simulink library "tramontina_database_xsenslib"  (R2023b)
settings: Solver=VariableStepAuto  StartTime=0.0  StopTime=10.0  RelTol=1e-3
libraries: canmsglib x46, simulink x1
(part 2 of 2)

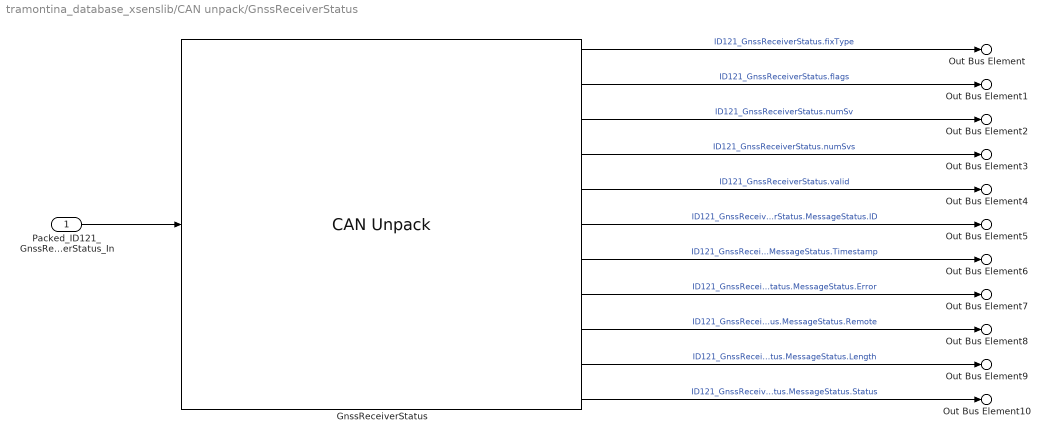
== system tramontina_database_xsenslib/CAN unpack/GnssReceiverStatus ==
  Packed_ID121_GnssReceiverStatus_In : Inport
  GnssReceiverStatus : canmsglib/CAN Unpack  CANdbFile=C:\Users\matlab.cut\Desktop\AMR\canbus_files\tramontina_database_xsens.dbc  MsgList=GnssReceiverStatus  MsgName=GnssReceiverStatus  MsgIDType=Standard (11-bit identifier)  MsgIdentifier=121  MsgLength=5  SignalInfo={'fixType','0','8','BE','unsigned','Standard','0','1','0','-Inf','Inf';'flags','16','8','BE','unsigned','Standard','0','1','0','-Inf','Inf';'numSv','8','8','BE','unsigned','Standard','0','1','0','-Inf','Inf';'numSvs','32','8','BE','unsigned','Standard','0','1','1','-Inf','Inf';'valid','24','8','BE','unsigned','Standard','0','1','0','-Inf','Inf'}  IDPort=on  TimestampPort=on  ErrorPort=on  RemotePort=on  LengthPort=on  StatusPort=on  ApplyMinMax=off
  Out Bus Element : Outport  PortName=ID121_GnssReceiverStatus  Element=fixType
  Out Bus Element1 : Outport  PortName=ID121_GnssReceiverStatus  Element=flags
  Out Bus Element2 : Outport  PortName=ID121_GnssReceiverStatus  Element=numSv
  Out Bus Element3 : Outport  PortName=ID121_GnssReceiverStatus  Element=numSvs
  Out Bus Element4 : Outport  PortName=ID121_GnssReceiverStatus  Element=valid
  Out Bus Element5 : Outport  PortName=ID121_GnssReceiverStatus  Element=MessageStatus.ID
  Out Bus Element6 : Outport  PortName=ID121_GnssReceiverStatus  Element=MessageStatus.Timestamp
  Out Bus Element7 : Outport  PortName=ID121_GnssReceiverStatus  Element=MessageStatus.Error
  Out Bus Element8 : Outport  PortName=ID121_GnssReceiverStatus  Element=MessageStatus.Remote
  Out Bus Element9 : Outport  PortName=ID121_GnssReceiverStatus  Element=MessageStatus.Length
  Out Bus Element10 : Outport  PortName=ID121_GnssReceiverStatus  Element=MessageStatus.Status
  wires:
  Packed_ID121_GnssReceiverStatus_In/1 -> GnssReceiverStatus/1
  GnssReceiverStatus/1 -> Out Bus Element/1  "ID121_GnssReceiverStatus.fixType"
  GnssReceiverStatus/2 -> Out Bus Element1/1  "ID121_GnssReceiverStatus.flags"
  GnssReceiverStatus/3 -> Out Bus Element2/1  "ID121_GnssReceiverStatus.numSv"
  GnssReceiverStatus/4 -> Out Bus Element3/1  "ID121_GnssReceiverStatus.numSvs"
  GnssReceiverStatus/5 -> Out Bus Element4/1  "ID121_GnssReceiverStatus.valid"
  GnssReceiverStatus/6 -> Out Bus Element5/1  "ID121_GnssReceiverStatus.MessageStatus.ID"
  GnssReceiverStatus/7 -> Out Bus Element6/1  "ID121_GnssReceiverStatus.MessageStatus.Timestamp"
  GnssReceiverStatus/8 -> Out Bus Element7/1  "ID121_GnssReceiverStatus.MessageStatus.Error"
  GnssReceiverStatus/9 -> Out Bus Element8/1  "ID121_GnssReceiverStatus.MessageStatus.Remote"
  GnssReceiverStatus/10 -> Out Bus Element9/1  "ID121_GnssReceiverStatus.MessageStatus.Length"
  GnssReceiverStatus/11 -> Out Bus Element10/1  "ID121_GnssReceiverStatus.MessageStatus.Status"

== system tramontina_database_xsenslib/CAN unpack/GroupCounter ==
  Packed_ID6_GroupCounter_In : Inport
  GroupCounter : canmsglib/CAN Unpack  CANdbFile=C:\Users\matlab.cut\Desktop\AMR\canbus_files\tramontina_database_xsens.dbc  MsgList=GroupCounter  MsgName=GroupCounter  MsgIDType=Standard (11-bit identifier)  MsgIdentifier=6  MsgLength=2  SignalInfo={'Counter','8','16','BE','unsigned','Standard','0','1','0','-Inf','Inf'}  IDPort=on  TimestampPort=on  ErrorPort=on  RemotePort=on  LengthPort=on  StatusPort=on  ApplyMinMax=off
  Out Bus Element : Outport  PortName=ID6_GroupCounter  Element=Counter
  Out Bus Element1 : Outport  PortName=ID6_GroupCounter  Element=MessageStatus.ID
  Out Bus Element2 : Outport  PortName=ID6_GroupCounter  Element=MessageStatus.Timestamp
  Out Bus Element3 : Outport  PortName=ID6_GroupCounter  Element=MessageStatus.Error
  Out Bus Element4 : Outport  PortName=ID6_GroupCounter  Element=MessageStatus.Remote
  Out Bus Element5 : Outport  PortName=ID6_GroupCounter  Element=MessageStatus.Length
  Out Bus Element6 : Outport  PortName=ID6_GroupCounter  Element=MessageStatus.Status
  wires:
  Packed_ID6_GroupCounter_In/1 -> GroupCounter/1
  GroupCounter/1 -> Out Bus Element/1  "ID6_GroupCounter.Counter"
  GroupCounter/2 -> Out Bus Element1/1  "ID6_GroupCounter.MessageStatus.ID"
  GroupCounter/3 -> Out Bus Element2/1  "ID6_GroupCounter.MessageStatus.Timestamp"
  GroupCounter/4 -> Out Bus Element3/1  "ID6_GroupCounter.MessageStatus.Error"
  GroupCounter/5 -> Out Bus Element4/1  "ID6_GroupCounter.MessageStatus.Remote"
  GroupCounter/6 -> Out Bus Element5/1  "ID6_GroupCounter.MessageStatus.Length"
  GroupCounter/7 -> Out Bus Element6/1  "ID6_GroupCounter.MessageStatus.Status"

== system tramontina_database_xsenslib/CAN unpack/LongLat ==
  Packed_ID113_LongLat_In : Inport
  LongLat : canmsglib/CAN Unpack  CANdbFile=C:\Users\matlab.cut\Desktop\AMR\canbus_files\tramontina_database_xsens.dbc  MsgList=LongLat  MsgName=LongLat  MsgIDType=Standard (11-bit identifier)  MsgIdentifier=113  MsgLength=8  SignalInfo={'latitude','24','32','BE','signed','Standard','0','5.9605e-08','0','-90','90';'longitude','56','32','BE','signed','Standard','0','1.1921e-07','0','-180','180'}  IDPort=on  TimestampPort=on  ErrorPort=on  RemotePort=on  LengthPort=on  StatusPort=on  ApplyMinMax=off
  Out Bus Element : Outport  PortName=ID113_LongLat  Element=latitude
  Out Bus Element1 : Outport  PortName=ID113_LongLat  Element=longitude
  Out Bus Element2 : Outport  PortName=ID113_LongLat  Element=MessageStatus.ID
  Out Bus Element3 : Outport  PortName=ID113_LongLat  Element=MessageStatus.Timestamp
  Out Bus Element4 : Outport  PortName=ID113_LongLat  Element=MessageStatus.Error
  Out Bus Element5 : Outport  PortName=ID113_LongLat  Element=MessageStatus.Remote
  Out Bus Element6 : Outport  PortName=ID113_LongLat  Element=MessageStatus.Length
  Out Bus Element7 : Outport  PortName=ID113_LongLat  Element=MessageStatus.Status
  wires:
  Packed_ID113_LongLat_In/1 -> LongLat/1
  LongLat/1 -> Out Bus Element/1  "ID113_LongLat.latitude"
  LongLat/2 -> Out Bus Element1/1  "ID113_LongLat.longitude"
  LongLat/3 -> Out Bus Element2/1  "ID113_LongLat.MessageStatus.ID"
  LongLat/4 -> Out Bus Element3/1  "ID113_LongLat.MessageStatus.Timestamp"
  LongLat/5 -> Out Bus Element4/1  "ID113_LongLat.MessageStatus.Error"
  LongLat/6 -> Out Bus Element5/1  "ID113_LongLat.MessageStatus.Remote"
  LongLat/7 -> Out Bus Element6/1  "ID113_LongLat.MessageStatus.Length"
  LongLat/8 -> Out Bus Element7/1  "ID113_LongLat.MessageStatus.Status"

== system tramontina_database_xsenslib/CAN unpack/MagneticField ==
  Packed_ID65_MagneticField_In : Inport
  MagneticField : canmsglib/CAN Unpack  CANdbFile=C:\Users\matlab.cut\Desktop\AMR\canbus_files\tramontina_database_xsens.dbc  MsgList=MagneticField  MsgName=MagneticField  MsgIDType=Standard (11-bit identifier)  MsgIdentifier=65  MsgLength=6  SignalInfo={'magX','8','16','BE','signed','Standard','0','0.00097656','0','-32','32';'magY','24','16','BE','signed','Standard','0','0.00097656','0','-32','32';'magZ','40','16','BE','signed','Standard','0','0.00097656','0','-32','32'}  IDPort=on  TimestampPort=on  ErrorPort=on  RemotePort=on  LengthPort=on  StatusPort=on  ApplyMinMax=off
  Out Bus Element : Outport  PortName=ID65_MagneticField  Element=magX
  Out Bus Element1 : Outport  PortName=ID65_MagneticField  Element=magY
  Out Bus Element2 : Outport  PortName=ID65_MagneticField  Element=magZ
  Out Bus Element3 : Outport  PortName=ID65_MagneticField  Element=MessageStatus.ID
  Out Bus Element4 : Outport  PortName=ID65_MagneticField  Element=MessageStatus.Timestamp
  Out Bus Element5 : Outport  PortName=ID65_MagneticField  Element=MessageStatus.Error
  Out Bus Element6 : Outport  PortName=ID65_MagneticField  Element=MessageStatus.Remote
  Out Bus Element7 : Outport  PortName=ID65_MagneticField  Element=MessageStatus.Length
  Out Bus Element8 : Outport  PortName=ID65_MagneticField  Element=MessageStatus.Status
  wires:
  Packed_ID65_MagneticField_In/1 -> MagneticField/1
  MagneticField/1 -> Out Bus Element/1  "ID65_MagneticField.magX"
  MagneticField/2 -> Out Bus Element1/1  "ID65_MagneticField.magY"
  MagneticField/3 -> Out Bus Element2/1  "ID65_MagneticField.magZ"
  MagneticField/4 -> Out Bus Element3/1  "ID65_MagneticField.MessageStatus.ID"
  MagneticField/5 -> Out Bus Element4/1  "ID65_MagneticField.MessageStatus.Timestamp"
  MagneticField/6 -> Out Bus Element5/1  "ID65_MagneticField.MessageStatus.Error"
  MagneticField/7 -> Out Bus Element6/1  "ID65_MagneticField.MessageStatus.Remote"
  MagneticField/8 -> Out Bus Element7/1  "ID65_MagneticField.MessageStatus.Length"
  MagneticField/9 -> Out Bus Element8/1  "ID65_MagneticField.MessageStatus.Status"

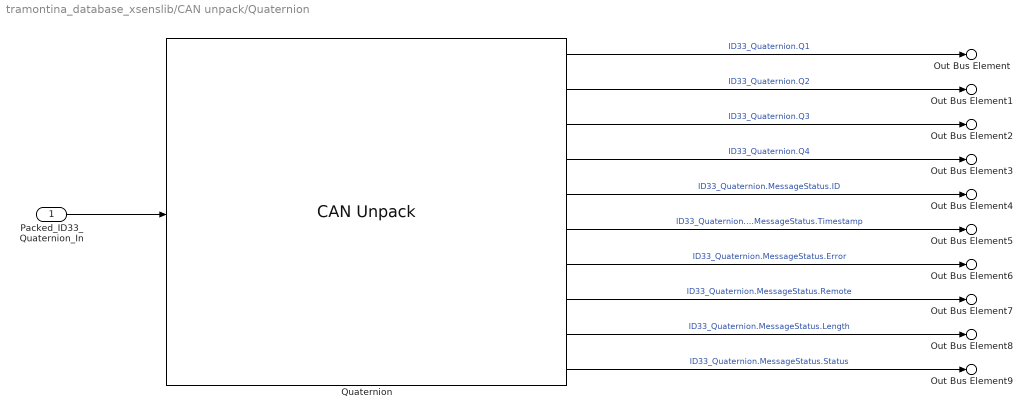
== system tramontina_database_xsenslib/CAN unpack/Quaternion ==
  Packed_ID33_Quaternion_In : Inport
  Quaternion : canmsglib/CAN Unpack  CANdbFile=C:\Users\matlab.cut\Desktop\AMR\canbus_files\tramontina_database_xsens.dbc  MsgList=Quaternion  MsgName=Quaternion  MsgIDType=Standard (11-bit identifier)  MsgIdentifier=33  MsgLength=8  SignalInfo={'Q1','8','16','BE','signed','Standard','0','3.0518e-05','0','-1','1';'Q2','24','16','BE','signed','Standard','0','3.0518e-05','0','-1','1';'Q3','40','16','BE','signed','Standard','0','3.0518e-05','0','-1','1';'Q4','56','16','BE','signed','Standard','0','3.0518e-05','0','-Inf','Inf'}  IDPort=on  TimestampPort=on  ErrorPort=on  RemotePort=on  LengthPort=on  StatusPort=on  ApplyMinMax=off
  Out Bus Element : Outport  PortName=ID33_Quaternion  Element=Q1
  Out Bus Element1 : Outport  PortName=ID33_Quaternion  Element=Q2
  Out Bus Element2 : Outport  PortName=ID33_Quaternion  Element=Q3
  Out Bus Element3 : Outport  PortName=ID33_Quaternion  Element=Q4
  Out Bus Element4 : Outport  PortName=ID33_Quaternion  Element=MessageStatus.ID
  Out Bus Element5 : Outport  PortName=ID33_Quaternion  Element=MessageStatus.Timestamp
  Out Bus Element6 : Outport  PortName=ID33_Quaternion  Element=MessageStatus.Error
  Out Bus Element7 : Outport  PortName=ID33_Quaternion  Element=MessageStatus.Remote
  Out Bus Element8 : Outport  PortName=ID33_Quaternion  Element=MessageStatus.Length
  Out Bus Element9 : Outport  PortName=ID33_Quaternion  Element=MessageStatus.Status
  wires:
  Packed_ID33_Quaternion_In/1 -> Quaternion/1
  Quaternion/1 -> Out Bus Element/1  "ID33_Quaternion.Q1"
  Quaternion/2 -> Out Bus Element1/1  "ID33_Quaternion.Q2"
  Quaternion/3 -> Out Bus Element2/1  "ID33_Quaternion.Q3"
  Quaternion/4 -> Out Bus Element3/1  "ID33_Quaternion.Q4"
  Quaternion/5 -> Out Bus Element4/1  "ID33_Quaternion.MessageStatus.ID"
  Quaternion/6 -> Out Bus Element5/1  "ID33_Quaternion.MessageStatus.Timestamp"
  Quaternion/7 -> Out Bus Element6/1  "ID33_Quaternion.MessageStatus.Error"
  Quaternion/8 -> Out Bus Element7/1  "ID33_Quaternion.MessageStatus.Remote"
  Quaternion/9 -> Out Bus Element8/1  "ID33_Quaternion.MessageStatus.Length"
  Quaternion/10 -> Out Bus Element9/1  "ID33_Quaternion.MessageStatus.Status"

== system tramontina_database_xsenslib/CAN unpack/RateOfTurn ==
  Packed_ID50_RateOfTurn_In : Inport
  RateOfTurn : canmsglib/CAN Unpack  CANdbFile=C:\Users\matlab.cut\Desktop\AMR\canbus_files\tramontina_database_xsens.dbc  MsgList=RateOfTurn  MsgName=RateOfTurn  MsgIDType=Standard (11-bit identifier)  MsgIdentifier=50  MsgLength=6  SignalInfo={'gyrX','8','16','BE','signed','Standard','0','0.0019531','0','-Inf','Inf';'gyrY','24','16','BE','signed','Standard','0','0.0019531','0','-Inf','Inf';'gyrZ','40','16','BE','signed','Standard','0','0.0019531','0','-Inf','Inf'}  IDPort=on  TimestampPort=on  ErrorPort=on  RemotePort=on  LengthPort=on  StatusPort=on  ApplyMinMax=off
  Out Bus Element : Outport  PortName=ID50_RateOfTurn  Element=gyrX
  Out Bus Element1 : Outport  PortName=ID50_RateOfTurn  Element=gyrY
  Out Bus Element2 : Outport  PortName=ID50_RateOfTurn  Element=gyrZ
  Out Bus Element3 : Outport  PortName=ID50_RateOfTurn  Element=MessageStatus.ID
  Out Bus Element4 : Outport  PortName=ID50_RateOfTurn  Element=MessageStatus.Timestamp
  Out Bus Element5 : Outport  PortName=ID50_RateOfTurn  Element=MessageStatus.Error
  Out Bus Element6 : Outport  PortName=ID50_RateOfTurn  Element=MessageStatus.Remote
  Out Bus Element7 : Outport  PortName=ID50_RateOfTurn  Element=MessageStatus.Length
  Out Bus Element8 : Outport  PortName=ID50_RateOfTurn  Element=MessageStatus.Status
  wires:
  Packed_ID50_RateOfTurn_In/1 -> RateOfTurn/1
  RateOfTurn/1 -> Out Bus Element/1  "ID50_RateOfTurn.gyrX"
  RateOfTurn/2 -> Out Bus Element1/1  "ID50_RateOfTurn.gyrY"
  RateOfTurn/3 -> Out Bus Element2/1  "ID50_RateOfTurn.gyrZ"
  RateOfTurn/4 -> Out Bus Element3/1  "ID50_RateOfTurn.MessageStatus.ID"
  RateOfTurn/5 -> Out Bus Element4/1  "ID50_RateOfTurn.MessageStatus.Timestamp"
  RateOfTurn/6 -> Out Bus Element5/1  "ID50_RateOfTurn.MessageStatus.Error"
  RateOfTurn/7 -> Out Bus Element6/1  "ID50_RateOfTurn.MessageStatus.Remote"
  RateOfTurn/8 -> Out Bus Element7/1  "ID50_RateOfTurn.MessageStatus.Length"
  RateOfTurn/9 -> Out Bus Element8/1  "ID50_RateOfTurn.MessageStatus.Status"

== system tramontina_database_xsenslib/CAN unpack/RateOfTurnHR ==
  Packed_ID97_RateOfTurnHR_In : Inport
  RateOfTurnHR : canmsglib/CAN Unpack  CANdbFile=C:\Users\matlab.cut\Desktop\AMR\canbus_files\tramontina_database_xsens.dbc  MsgList=RateOfTurnHR  MsgName=RateOfTurnHR  MsgIDType=Standard (11-bit identifier)  MsgIdentifier=97  MsgLength=6  SignalInfo={'HrGyrX','8','16','BE','signed','Standard','0','0.0019531','0','-Inf','Inf';'HrGyrY','24','16','BE','signed','Standard','0','0.0019531','0','-Inf','Inf';'HrGyrZ','40','16','BE','signed','Standard','0','0.0019531','0','-Inf','Inf'}  IDPort=on  TimestampPort=on  ErrorPort=on  RemotePort=on  LengthPort=on  StatusPort=on  ApplyMinMax=off
  Out Bus Element : Outport  PortName=ID97_RateOfTurnHR  Element=HrGyrX
  Out Bus Element1 : Outport  PortName=ID97_RateOfTurnHR  Element=HrGyrY
  Out Bus Element2 : Outport  PortName=ID97_RateOfTurnHR  Element=HrGyrZ
  Out Bus Element3 : Outport  PortName=ID97_RateOfTurnHR  Element=MessageStatus.ID
  Out Bus Element4 : Outport  PortName=ID97_RateOfTurnHR  Element=MessageStatus.Timestamp
  Out Bus Element5 : Outport  PortName=ID97_RateOfTurnHR  Element=MessageStatus.Error
  Out Bus Element6 : Outport  PortName=ID97_RateOfTurnHR  Element=MessageStatus.Remote
  Out Bus Element7 : Outport  PortName=ID97_RateOfTurnHR  Element=MessageStatus.Length
  Out Bus Element8 : Outport  PortName=ID97_RateOfTurnHR  Element=MessageStatus.Status
  wires:
  Packed_ID97_RateOfTurnHR_In/1 -> RateOfTurnHR/1
  RateOfTurnHR/1 -> Out Bus Element/1  "ID97_RateOfTurnHR.HrGyrX"
  RateOfTurnHR/2 -> Out Bus Element1/1  "ID97_RateOfTurnHR.HrGyrY"
  RateOfTurnHR/3 -> Out Bus Element2/1  "ID97_RateOfTurnHR.HrGyrZ"
  RateOfTurnHR/4 -> Out Bus Element3/1  "ID97_RateOfTurnHR.MessageStatus.ID"
  RateOfTurnHR/5 -> Out Bus Element4/1  "ID97_RateOfTurnHR.MessageStatus.Timestamp"
  RateOfTurnHR/6 -> Out Bus Element5/1  "ID97_RateOfTurnHR.MessageStatus.Error"
  RateOfTurnHR/7 -> Out Bus Element6/1  "ID97_RateOfTurnHR.MessageStatus.Remote"
  RateOfTurnHR/8 -> Out Bus Element7/1  "ID97_RateOfTurnHR.MessageStatus.Length"
  RateOfTurnHR/9 -> Out Bus Element8/1  "ID97_RateOfTurnHR.MessageStatus.Status"

== system tramontina_database_xsenslib/CAN unpack/SampleTime ==
  Packed_ID5_SampleTime_In : Inport
  SampleTime : canmsglib/CAN Unpack  CANdbFile=C:\Users\matlab.cut\Desktop\AMR\canbus_files\tramontina_database_xsens.dbc  MsgList=SampleTime  MsgName=SampleTime  MsgIDType=Standard (11-bit identifier)  MsgIdentifier=5  MsgLength=4  SignalInfo={'Timestamp','24','32','BE','unsigned','Standard','0','1','0','-Inf','Inf'}  IDPort=on  TimestampPort=on  ErrorPort=on  RemotePort=on  LengthPort=on  StatusPort=on  ApplyMinMax=off
  Out Bus Element : Outport  PortName=ID5_SampleTime  Element=Timestamp
  Out Bus Element1 : Outport  PortName=ID5_SampleTime  Element=MessageStatus.ID
  Out Bus Element2 : Outport  PortName=ID5_SampleTime  Element=MessageStatus.Timestamp
  Out Bus Element3 : Outport  PortName=ID5_SampleTime  Element=MessageStatus.Error
  Out Bus Element4 : Outport  PortName=ID5_SampleTime  Element=MessageStatus.Remote
  Out Bus Element5 : Outport  PortName=ID5_SampleTime  Element=MessageStatus.Length
  Out Bus Element6 : Outport  PortName=ID5_SampleTime  Element=MessageStatus.Status
  wires:
  Packed_ID5_SampleTime_In/1 -> SampleTime/1
  SampleTime/1 -> Out Bus Element/1  "ID5_SampleTime.Timestamp"
  SampleTime/2 -> Out Bus Element1/1  "ID5_SampleTime.MessageStatus.ID"
  SampleTime/3 -> Out Bus Element2/1  "ID5_SampleTime.MessageStatus.Timestamp"
  SampleTime/4 -> Out Bus Element3/1  "ID5_SampleTime.MessageStatus.Error"
  SampleTime/5 -> Out Bus Element4/1  "ID5_SampleTime.MessageStatus.Remote"
  SampleTime/6 -> Out Bus Element5/1  "ID5_SampleTime.MessageStatus.Length"
  SampleTime/7 -> Out Bus Element6/1  "ID5_SampleTime.MessageStatus.Status"

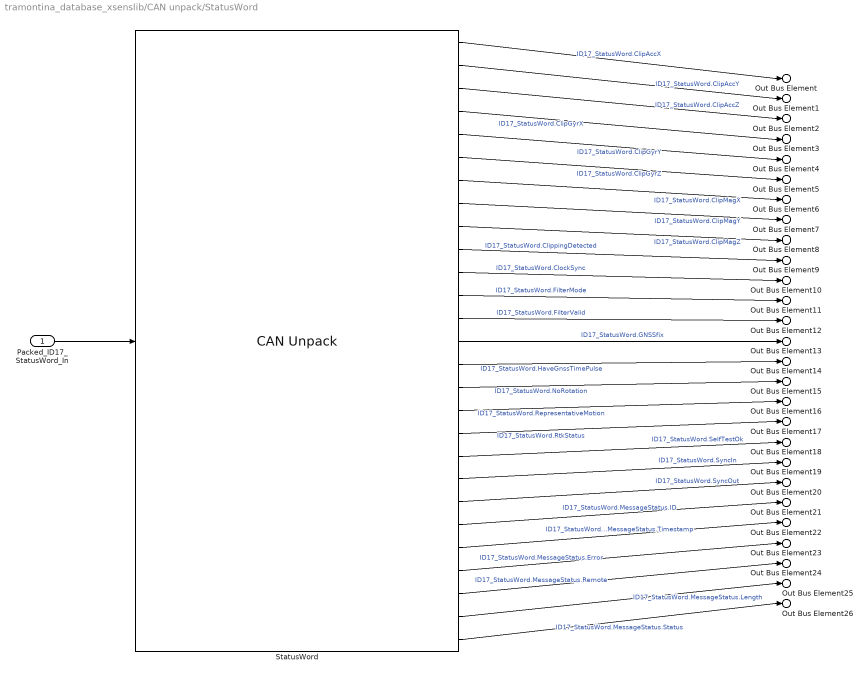
== system tramontina_database_xsenslib/CAN unpack/StatusWord ==
  Packed_ID17_StatusWord_In : Inport
  StatusWord : canmsglib/CAN Unpack  CANdbFile=C:\Users\matlab.cut\Desktop\AMR\canbus_files\tramontina_database_xsens.dbc  MsgList=StatusWord  MsgName=StatusWord  MsgIDType=Standard (11-bit identifier)  MsgIdentifier=17  MsgLength=4  SignalInfo={'ClipAccX','16','1','LE','unsigned','Standard','0','1','0','0','1';'ClipAccY','17','1','LE','unsigned','Standard','0','1','0','0','1';'ClipAccZ','18','1','LE','unsigned','Standard','0','1','0','0','1';'ClipGyrX','19','1','LE','unsigned','Standard','0','1','0','0','1';'ClipGyrY','20','1','LE','unsigned','Standard','0','1','0','0','1';'ClipGyrZ','21','1','LE','unsigned','Standard','0','1','0','0','1';'ClipMagX','22','1','LE','unsigned','Standard','0','1','0','0','1';'ClipMagY','23','1','LE','unsigned','Standard','0','1','0','0','1';'ClipMagZ','8','1','LE','unsigned','Standard','0','1','0','0','1';'ClippingDetected','11','1','LE','unsigned','Standard','0','1','0','0','1';'ClockSync','30','1','LE','unsigned','Standard','0','1','0','0','1';'FilterMode','15','3','BE','unsigned','Standard','0','1','0','-Inf','Inf';'FilterValid','25','1','LE','unsigned','Standard','0','1','0','0','1';'GNSSfix','26','1','LE','unsigned','Standard','0','1','0','0','1';'HaveGnssTimePulse','2','1','LE','unsigned','Standard','0','1','0','0','1';'NoRotation','27','2','BE','unsigned','Standard','0','1','0','0','3';'RepresentativeMotion','29','1','LE','unsigned','Standard','0','1','0','0','1';'RtkStatus','3','2','BE','unsigned','Standard','0','1','0','0','1';'SelfTestOk','24','1','LE','unsigned','Standard','0','1','0','0','1';'SyncIn','13','1','LE','unsigned','Standard','0','1','0','0','1';'SyncOut','14','1','LE','unsigned','Standard','0','1','0','0','1'}  IDPort=on  TimestampPort=on  ErrorPort=on  RemotePort=on  LengthPort=on  StatusPort=on  ApplyMinMax=off
  Out Bus Element : Outport  PortName=ID17_StatusWord  Element=ClipAccX
  Out Bus Element1 : Outport  PortName=ID17_StatusWord  Element=ClipAccY
  Out Bus Element2 : Outport  PortName=ID17_StatusWord  Element=ClipAccZ
  Out Bus Element3 : Outport  PortName=ID17_StatusWord  Element=ClipGyrX
  Out Bus Element4 : Outport  PortName=ID17_StatusWord  Element=ClipGyrY
  Out Bus Element5 : Outport  PortName=ID17_StatusWord  Element=ClipGyrZ
  Out Bus Element6 : Outport  PortName=ID17_StatusWord  Element=ClipMagX
  Out Bus Element7 : Outport  PortName=ID17_StatusWord  Element=ClipMagY
  Out Bus Element8 : Outport  PortName=ID17_StatusWord  Element=ClipMagZ
  Out Bus Element9 : Outport  PortName=ID17_StatusWord  Element=ClippingDetected
  Out Bus Element10 : Outport  PortName=ID17_StatusWord  Element=ClockSync
  Out Bus Element11 : Outport  PortName=ID17_StatusWord  Element=FilterMode
  Out Bus Element12 : Outport  PortName=ID17_StatusWord  Element=FilterValid
  Out Bus Element13 : Outport  PortName=ID17_StatusWord  Element=GNSSfix
  Out Bus Element14 : Outport  PortName=ID17_StatusWord  Element=HaveGnssTimePulse
  Out Bus Element15 : Outport  PortName=ID17_StatusWord  Element=NoRotation
  Out Bus Element16 : Outport  PortName=ID17_StatusWord  Element=RepresentativeMotion
  Out Bus Element17 : Outport  PortName=ID17_StatusWord  Element=RtkStatus
  Out Bus Element18 : Outport  PortName=ID17_StatusWord  Element=SelfTestOk
  Out Bus Element19 : Outport  PortName=ID17_StatusWord  Element=SyncIn
  Out Bus Element20 : Outport  PortName=ID17_StatusWord  Element=SyncOut
  Out Bus Element21 : Outport  PortName=ID17_StatusWord  Element=MessageStatus.ID
  Out Bus Element22 : Outport  PortName=ID17_StatusWord  Element=MessageStatus.Timestamp
  Out Bus Element23 : Outport  PortName=ID17_StatusWord  Element=MessageStatus.Error
  Out Bus Element24 : Outport  PortName=ID17_StatusWord  Element=MessageStatus.Remote
  Out Bus Element25 : Outport  PortName=ID17_StatusWord  Element=MessageStatus.Length
  Out Bus Element26 : Outport  PortName=ID17_StatusWord  Element=MessageStatus.Status
  wires:
  Packed_ID17_StatusWord_In/1 -> StatusWord/1
  StatusWord/1 -> Out Bus Element/1  "ID17_StatusWord.ClipAccX"
  StatusWord/2 -> Out Bus Element1/1  "ID17_StatusWord.ClipAccY"
  StatusWord/3 -> Out Bus Element2/1  "ID17_StatusWord.ClipAccZ"
  StatusWord/4 -> Out Bus Element3/1  "ID17_StatusWord.ClipGyrX"
  StatusWord/5 -> Out Bus Element4/1  "ID17_StatusWord.ClipGyrY"
  StatusWord/6 -> Out Bus Element5/1  "ID17_StatusWord.ClipGyrZ"
  StatusWord/7 -> Out Bus Element6/1  "ID17_StatusWord.ClipMagX"
  StatusWord/8 -> Out Bus Element7/1  "ID17_StatusWord.ClipMagY"
  StatusWord/9 -> Out Bus Element8/1  "ID17_StatusWord.ClipMagZ"
  StatusWord/10 -> Out Bus Element9/1  "ID17_StatusWord.ClippingDetected"
  StatusWord/11 -> Out Bus Element10/1  "ID17_StatusWord.ClockSync"
  StatusWord/12 -> Out Bus Element11/1  "ID17_StatusWord.FilterMode"
  StatusWord/13 -> Out Bus Element12/1  "ID17_StatusWord.FilterValid"
  StatusWord/14 -> Out Bus Element13/1  "ID17_StatusWord.GNSSfix"
  StatusWord/15 -> Out Bus Element14/1  "ID17_StatusWord.HaveGnssTimePulse"
  StatusWord/16 -> Out Bus Element15/1  "ID17_StatusWord.NoRotation"
  StatusWord/17 -> Out Bus Element16/1  "ID17_StatusWord.RepresentativeMotion"
  StatusWord/18 -> Out Bus Element17/1  "ID17_StatusWord.RtkStatus"
  StatusWord/19 -> Out Bus Element18/1  "ID17_StatusWord.SelfTestOk"
  StatusWord/20 -> Out Bus Element19/1  "ID17_StatusWord.SyncIn"
  StatusWord/21 -> Out Bus Element20/1  "ID17_StatusWord.SyncOut"
  StatusWord/22 -> Out Bus Element21/1  "ID17_StatusWord.MessageStatus.ID"
  StatusWord/23 -> Out Bus Element22/1  "ID17_StatusWord.MessageStatus.Timestamp"
  StatusWord/24 -> Out Bus Element23/1  "ID17_StatusWord.MessageStatus.Error"
  StatusWord/25 -> Out Bus Element24/1  "ID17_StatusWord.MessageStatus.Remote"
  StatusWord/26 -> Out Bus Element25/1  "ID17_StatusWord.MessageStatus.Length"
  StatusWord/27 -> Out Bus Element26/1  "ID17_StatusWord.MessageStatus.Status"

== system tramontina_database_xsenslib/CAN unpack/Temperature ==
  Packed_ID81_Temperature_In : Inport
  Temperature : canmsglib/CAN Unpack  CANdbFile=C:\Users\matlab.cut\Desktop\AMR\canbus_files\tramontina_database_xsens.dbc  MsgList=Temperature  MsgName=Temperature  MsgIDType=Standard (11-bit identifier)  MsgIdentifier=81  MsgLength=2  SignalInfo={'Temperature','8','16','BE','signed','Standard','0','0.0039062','0','-40','85'}  IDPort=on  TimestampPort=on  ErrorPort=on  RemotePort=on  LengthPort=on  StatusPort=on  ApplyMinMax=off
  Out Bus Element : Outport  PortName=ID81_Temperature  Element=Temperature
  Out Bus Element1 : Outport  PortName=ID81_Temperature  Element=MessageStatus.ID
  Out Bus Element2 : Outport  PortName=ID81_Temperature  Element=MessageStatus.Timestamp
  Out Bus Element3 : Outport  PortName=ID81_Temperature  Element=MessageStatus.Error
  Out Bus Element4 : Outport  PortName=ID81_Temperature  Element=MessageStatus.Remote
  Out Bus Element5 : Outport  PortName=ID81_Temperature  Element=MessageStatus.Length
  Out Bus Element6 : Outport  PortName=ID81_Temperature  Element=MessageStatus.Status
  wires:
  Packed_ID81_Temperature_In/1 -> Temperature/1
  Temperature/1 -> Out Bus Element/1  "ID81_Temperature.Temperature"
  Temperature/2 -> Out Bus Element1/1  "ID81_Temperature.MessageStatus.ID"
  Temperature/3 -> Out Bus Element2/1  "ID81_Temperature.MessageStatus.Timestamp"
  Temperature/4 -> Out Bus Element3/1  "ID81_Temperature.MessageStatus.Error"
  Temperature/5 -> Out Bus Element4/1  "ID81_Temperature.MessageStatus.Remote"
  Temperature/6 -> Out Bus Element5/1  "ID81_Temperature.MessageStatus.Length"
  Temperature/7 -> Out Bus Element6/1  "ID81_Temperature.MessageStatus.Status"

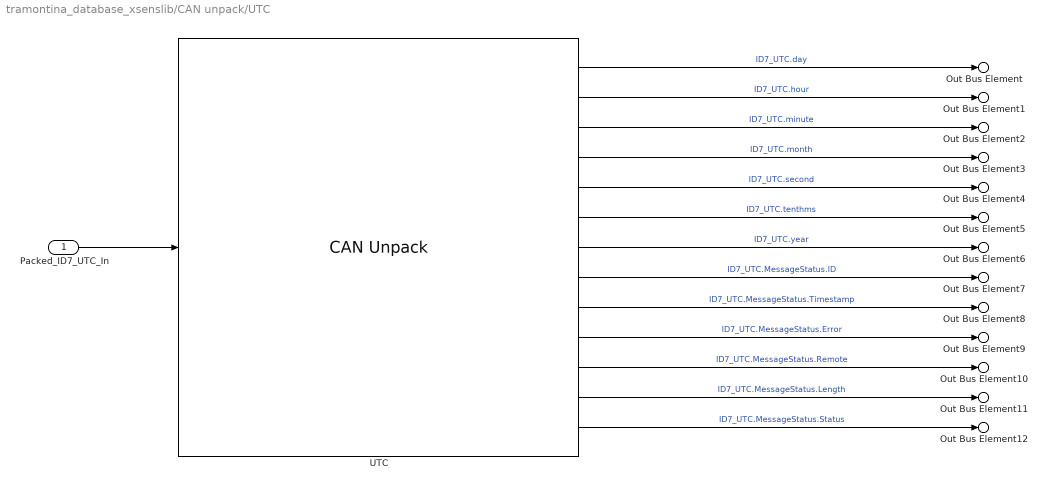
== system tramontina_database_xsenslib/CAN unpack/UTC ==
  Packed_ID7_UTC_In : Inport
  UTC : canmsglib/CAN Unpack  CANdbFile=C:\Users\matlab.cut\Desktop\AMR\canbus_files\tramontina_database_xsens.dbc  MsgList=UTC  MsgName=UTC  MsgIDType=Standard (11-bit identifier)  MsgIdentifier=7  MsgLength=8  SignalInfo={'day','16','8','BE','unsigned','Standard','0','1','0','1','31';'hour','24','8','BE','unsigned','Standard','0','1','0','0','24';'minute','32','8','BE','unsigned','Standard','0','1','0','0','60';'month','8','8','BE','unsigned','Standard','0','1','0','1','12';'second','40','8','BE','unsigned','Standard','0','1','0','0','60';'tenthms','56','16','BE','unsigned','Standard','0','1','0','-Inf','Inf';'year','0','8','BE','unsigned','Standard','0','1','0','-Inf','Inf'}  IDPort=on  TimestampPort=on  ErrorPort=on  RemotePort=on  LengthPort=on  StatusPort=on  ApplyMinMax=off
  Out Bus Element : Outport  PortName=ID7_UTC  Element=day
  Out Bus Element1 : Outport  PortName=ID7_UTC  Element=hour
  Out Bus Element2 : Outport  PortName=ID7_UTC  Element=minute
  Out Bus Element3 : Outport  PortName=ID7_UTC  Element=month
  Out Bus Element4 : Outport  PortName=ID7_UTC  Element=second
  Out Bus Element5 : Outport  PortName=ID7_UTC  Element=tenthms
  Out Bus Element6 : Outport  PortName=ID7_UTC  Element=year
  Out Bus Element7 : Outport  PortName=ID7_UTC  Element=MessageStatus.ID
  Out Bus Element8 : Outport  PortName=ID7_UTC  Element=MessageStatus.Timestamp
  Out Bus Element9 : Outport  PortName=ID7_UTC  Element=MessageStatus.Error
  Out Bus Element10 : Outport  PortName=ID7_UTC  Element=MessageStatus.Remote
  Out Bus Element11 : Outport  PortName=ID7_UTC  Element=MessageStatus.Length
  Out Bus Element12 : Outport  PortName=ID7_UTC  Element=MessageStatus.Status
  wires:
  Packed_ID7_UTC_In/1 -> UTC/1
  UTC/1 -> Out Bus Element/1  "ID7_UTC.day"
  UTC/2 -> Out Bus Element1/1  "ID7_UTC.hour"
  UTC/3 -> Out Bus Element2/1  "ID7_UTC.minute"
  UTC/4 -> Out Bus Element3/1  "ID7_UTC.month"
  UTC/5 -> Out Bus Element4/1  "ID7_UTC.second"
  UTC/6 -> Out Bus Element5/1  "ID7_UTC.tenthms"
  UTC/7 -> Out Bus Element6/1  "ID7_UTC.year"
  UTC/8 -> Out Bus Element7/1  "ID7_UTC.MessageStatus.ID"
  UTC/9 -> Out Bus Element8/1  "ID7_UTC.MessageStatus.Timestamp"
  UTC/10 -> Out Bus Element9/1  "ID7_UTC.MessageStatus.Error"
  UTC/11 -> Out Bus Element10/1  "ID7_UTC.MessageStatus.Remote"
  UTC/12 -> Out Bus Element11/1  "ID7_UTC.MessageStatus.Length"
  UTC/13 -> Out Bus Element12/1  "ID7_UTC.MessageStatus.Status"

== system tramontina_database_xsenslib/CAN unpack/Velocity ==
  Packed_ID118_Velocity_In : Inport
  Velocity : canmsglib/CAN Unpack  CANdbFile=C:\Users\matlab.cut\Desktop\AMR\canbus_files\tramontina_database_xsens.dbc  MsgList=Velocity  MsgName=Velocity  MsgIDType=Standard (11-bit identifier)  MsgIdentifier=118  MsgLength=6  SignalInfo={'velX','8','16','BE','signed','Standard','0','0.015625','0','-500','500';'velY','24','16','BE','signed','Standard','0','0.015625','0','-500','500';'velZ','40','16','BE','signed','Standard','0','0.015625','0','-500','500'}  IDPort=on  TimestampPort=on  ErrorPort=on  RemotePort=on  LengthPort=on  StatusPort=on  ApplyMinMax=off
  Out Bus Element : Outport  PortName=ID118_Velocity  Element=velX
  Out Bus Element1 : Outport  PortName=ID118_Velocity  Element=velY
  Out Bus Element2 : Outport  PortName=ID118_Velocity  Element=velZ
  Out Bus Element3 : Outport  PortName=ID118_Velocity  Element=MessageStatus.ID
  Out Bus Element4 : Outport  PortName=ID118_Velocity  Element=MessageStatus.Timestamp
  Out Bus Element5 : Outport  PortName=ID118_Velocity  Element=MessageStatus.Error
  Out Bus Element6 : Outport  PortName=ID118_Velocity  Element=MessageStatus.Remote
  Out Bus Element7 : Outport  PortName=ID118_Velocity  Element=MessageStatus.Length
  Out Bus Element8 : Outport  PortName=ID118_Velocity  Element=MessageStatus.Status
  wires:
  Packed_ID118_Velocity_In/1 -> Velocity/1
  Velocity/1 -> Out Bus Element/1  "ID118_Velocity.velX"
  Velocity/2 -> Out Bus Element1/1  "ID118_Velocity.velY"
  Velocity/3 -> Out Bus Element2/1  "ID118_Velocity.velZ"
  Velocity/4 -> Out Bus Element3/1  "ID118_Velocity.MessageStatus.ID"
  Velocity/5 -> Out Bus Element4/1  "ID118_Velocity.MessageStatus.Timestamp"
  Velocity/6 -> Out Bus Element5/1  "ID118_Velocity.MessageStatus.Error"
  Velocity/7 -> Out Bus Element6/1  "ID118_Velocity.MessageStatus.Remote"
  Velocity/8 -> Out Bus Element7/1  "ID118_Velocity.MessageStatus.Length"
  Velocity/9 -> Out Bus Element8/1  "ID118_Velocity.MessageStatus.Status"

== system tramontina_database_xsenslib/CAN unpack/Warning ==
  Packed_ID2_Warning_In : Inport
  Warning : canmsglib/CAN Unpack  CANdbFile=C:\Users\matlab.cut\Desktop\AMR\canbus_files\tramontina_database_xsens.dbc  MsgList=Warning  MsgName=Warning  MsgIDType=Standard (11-bit identifier)  MsgIdentifier=2  MsgLength=1  SignalInfo={'WarningCode','0','8','BE','unsigned','Standard','0','1','0','-Inf','Inf'}  IDPort=on  TimestampPort=on  ErrorPort=on  RemotePort=on  LengthPort=on  StatusPort=on  ApplyMinMax=off
  Out Bus Element : Outport  PortName=ID2_Warning  Element=WarningCode
  Out Bus Element1 : Outport  PortName=ID2_Warning  Element=MessageStatus.ID
  Out Bus Element2 : Outport  PortName=ID2_Warning  Element=MessageStatus.Timestamp
  Out Bus Element3 : Outport  PortName=ID2_Warning  Element=MessageStatus.Error
  Out Bus Element4 : Outport  PortName=ID2_Warning  Element=MessageStatus.Remote
  Out Bus Element5 : Outport  PortName=ID2_Warning  Element=MessageStatus.Length
  Out Bus Element6 : Outport  PortName=ID2_Warning  Element=MessageStatus.Status
  wires:
  Packed_ID2_Warning_In/1 -> Warning/1
  Warning/1 -> Out Bus Element/1  "ID2_Warning.WarningCode"
  Warning/2 -> Out Bus Element1/1  "ID2_Warning.MessageStatus.ID"
  Warning/3 -> Out Bus Element2/1  "ID2_Warning.MessageStatus.Timestamp"
  Warning/4 -> Out Bus Element3/1  "ID2_Warning.MessageStatus.Error"
  Warning/5 -> Out Bus Element4/1  "ID2_Warning.MessageStatus.Remote"
  Warning/6 -> Out Bus Element5/1  "ID2_Warning.MessageStatus.Length"
  Warning/7 -> Out Bus Element6/1  "ID2_Warning.MessageStatus.Status"
